simulink model "RoadTestingFinalVersionWitThreat"  (Simulink 7.6)
settings: Solver=ode3  StartTime=0.0  StopTime=19  FixedStep=.05  RelTol=1e-3
StartFcn:
  | Threshold = 12;
  | MaxCluster = 25;
  | Num_Beams = 726;
  | Road_Width = 9;
  | Cone_Area = 0.125;
  | Cone_Spacing = 4.45;
  | Scaling = 1.1;
  | areaBuffer = 0.125;
  | spacingBuffer = 0.05;
  | RoadfromConeoffset = 0.3;
  | threatThreshold = 65;
  | distThreshold = 10;
  | minSpeed = 2.0;
  | minDistance = 1.0;
  | threatConeAngle = 70;
  | allowableDistToCone = 1.25;
  | thresholdManueverAngle = 27.5;
  | maxStepSize = 1.0;
  | aspectRatioBuffer = 1;
  | javaaddpath({'/'});
  | import ClusterMethodWithVelocityThreat.*;
  | DataCluster = ClusterMethodWithVelocityThreat(Threshold,MaxCluster,Scaling,...
  | Road_Width,Cone_Area,Cone_Spacing,areaBuffer,spacingBuffer,RoadfromConeoffset,threatThreshold,...
  | distThreshold,minSpeed,minDistance,threatConeAngle,allowableDistToCone,thresholdManueverAngle,maxStepSize,aspectRatioBuffer);
  | %DataCluster = ClusterMethodWithRoad(Threshold,MaxCluster,Scaling,...
  | %Road_Width,Cone_Area,Cone_Spacing,areaBuffer,spacingBuffer,RoadfromConeoffset);
  | eml.extrinsic('evalin');
StopFcn:
  | clear DataCluster;
  | clear Threshold;
  | clear MaxCluster;
  | clear Num_Beams;
  | clear Road_Width;
  | clear Cone_Area;
  | clear Cone_Spacing;
  | clear Scaling;
  | clear areaBuffer;
  | clear spacingBuffer;
  | clear RoadfromConeoffset;
  | clear threatThreshold;
  | clear distThreshold;
  | clear minSpeed;
  | clear minDistance;
  | clear threatConeAngle;
  | clear allowableDistToCone;
  | clear thresholdManueverAngle;
  | clear maxStepSize;
  | clear aspectRatioBuffer;
settings Model: Creator=Thomas  LastModifiedBy=ipainter
settings DebuggingCC: FcnCallInpInsideContextMsg=Enable All

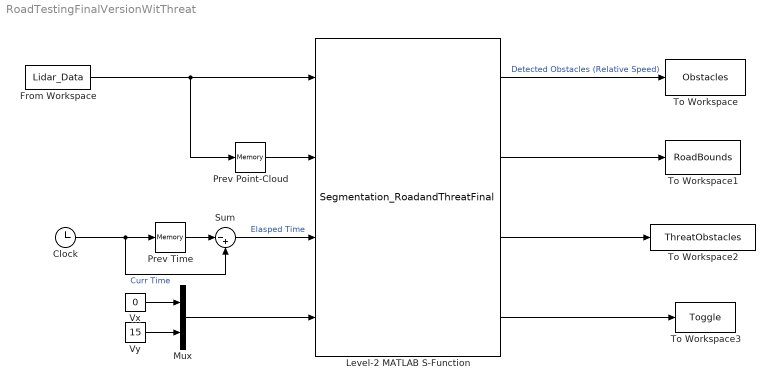
== system RoadTestingFinalVersionWitThreat ==
  Clock : Clock
      settings: Decimation=10
  From Workspace : FromWorkspace  VariableName=Lidar_Data  SampleTime=0  OutputAfterFinalValue=Setting to zero
  Level-2 MATLAB S-Function : M-S-Function  FunctionName=Segmentation_RoadandThreatFinal
  Mux : Mux  Inputs=2
  Prev Point-Cloud : Memory
  Prev Time : Memory
  Sum : Sum  Inputs=|-+
  To Workspace : ToWorkspace  VariableName=Obstacles  SampleTime=-1  SaveFormat=Structure With Time
  To Workspace1 : ToWorkspace  VariableName=RoadBounds  SampleTime=-1  SaveFormat=Structure With Time
  To Workspace2 : ToWorkspace  VariableName=ThreatObstacles  SampleTime=-1  SaveFormat=Structure With Time
  To Workspace3 : ToWorkspace  VariableName=Toggle  SampleTime=-1  SaveFormat=Structure With Time
  Vx : Constant  Value=0
  Vy : Constant  Value=15
  wires:
  Prev Time/1 -> Sum/1
  Sum/1 -> Level-2 MATLAB S-Function/3  "Elasped Time"
  Clock/1 -> Prev Time/1, Sum/2  "Curr Time"
  Prev Point-Cloud/1 -> Level-2 MATLAB S-Function/2
  Level-2 MATLAB S-Function/1 -> To Workspace/1  "Detected Obstacles (Relative Speed)"
  Level-2 MATLAB S-Function/2 -> To Workspace1/1
  Vx/1 -> Mux/1
  Vy/1 -> Mux/2
  From Workspace/1 -> Prev Point-Cloud/1, Level-2 MATLAB S-Function/1
  Mux/1 -> Level-2 MATLAB S-Function/4
  Level-2 MATLAB S-Function/3 -> To Workspace2/1
  Level-2 MATLAB S-Function/4 -> To Workspace3/1
